simulink model "UART"  (R2020a)
settings: Solver=VariableStepAuto  StartTime=0.0  StopTime=10.0  RelTol=1e-3
libraries: modelsimlib x2, simulink x1
settings Model: Creator=ADMIN  LastModifiedBy=ADMIN

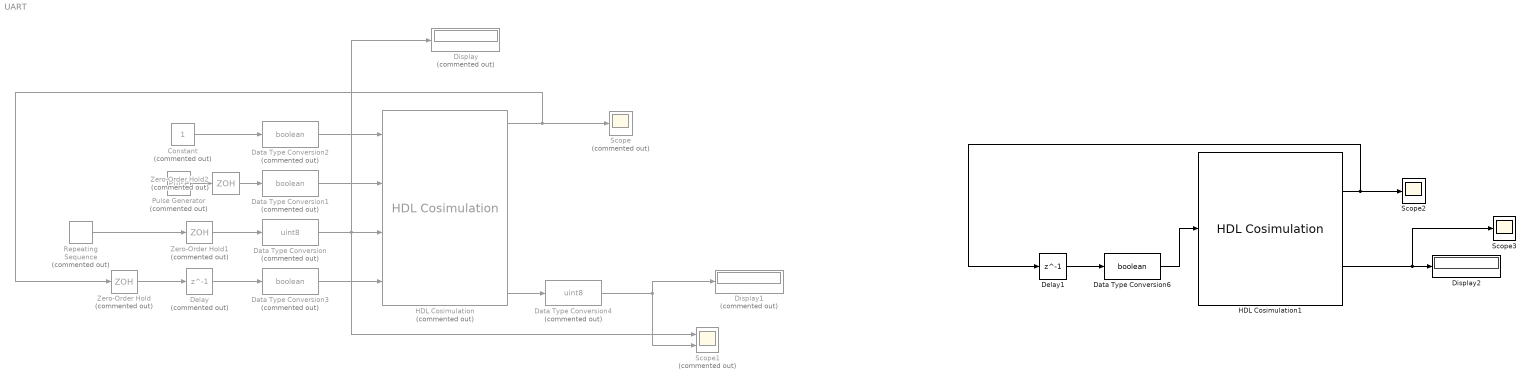
== system UART ==
  Constant : Constant  Commented=on
  Data Type Conversion : DataTypeConversion  Commented=on  OutDataTypeStr=uint8
  Data Type Conversion1 : DataTypeConversion  Commented=on  OutDataTypeStr=boolean
  Data Type Conversion2 : DataTypeConversion  Commented=on  OutDataTypeStr=boolean
  Data Type Conversion3 : DataTypeConversion  Commented=on  OutDataTypeStr=boolean
  Data Type Conversion4 : DataTypeConversion  Commented=on  OutDataTypeStr=uint8
  Data Type Conversion6 : DataTypeConversion  OutDataTypeStr=boolean
  Delay : Delay  Commented=on  DelayLength=1  SampleTime=2e-8
  Delay1 : Delay  DelayLength=1  SampleTime=2e-8
  Display : Display  Commented=on
      settings: Format=binary (Stored Integer)
  Display1 : Display  Commented=on
      settings: Format=binary (Stored Integer)
  Display2 : Display
      settings: Format=binary (Stored Integer)
  HDL Cosimulation : modelsimlib/HDL Cosimulation  Commented=on  PortPaths=/uart/RST_N;/uart/TX_ENA;/uart/TX_DATA;/uart/TX;/uart/TX_BUSY;/uart/TX_DONE;/uart/RX;/uart/RX_BUSY;/uart/RX_ERROR;/uart/RX_DATA  PortModes=[1 1 1 2 2 2 1 2 2 2 ]  PortTimes=[-1,-1,-1,2e-8,2e-8,2e-8,-1,2e-8,2e-8,2e-8]  PortSigns=[-1 -1 -1 -1 -1 -1 -1 -1 -1 -1 ]  PortFracLengths=[0,0,0,0,0,0,0,0,0,0]  CommLocal=on  CommSharedMemory=on  CommPortNumber=4449  CommShowInfo=on  ClockPaths=/uart/CLK  ClockModes=[2 ]  ClockTimes=[2e-8]  TclPreSimCommand="puts \"Running Simulink Cosimulation block.\""  TclPostSimCommand="puts \"done\""  TimingMode=s  TimingScaleFactor=1  idxCellArray={'UNUSED_VAR'}  CosimBypass=Full Simulation  AllowDirectFeedthrough=on  ProductName=EDA Simulator Link MQ  RunAutoTimescale=off  HdlClocks=0  PreRunTime=0  PreRunTimeUnit=ns
      settings: SourceProductBaseCode=ES
  HDL Cosimulation1 : modelsimlib/HDL Cosimulation  PortPaths=/transfer/TX;/transfer/RX;/transfer/RX_DATA  PortModes=[2 1 2 ]  PortTimes=[2e-8,-1,2e-8]  PortSigns=[-1 -1 -1 ]  PortFracLengths=[0,0,0]  CommLocal=on  CommSharedMemory=on  CommPortNumber=4449  CommShowInfo=on  ClockPaths=/transfer/CLK  ClockModes=[2 ]  ClockTimes=[2e-8]  TclPreSimCommand="puts \"Running Simulink Cosimulation block.\""  TclPostSimCommand="puts \"done\""  TimingMode=s  TimingScaleFactor=1  idxCellArray={'UNUSED_VAR'}  CosimBypass=Full Simulation  AllowDirectFeedthrough=on  ProductName=EDA Simulator Link MQ  RunAutoTimescale=off  HdlClocks=0  PreRunTime=0  PreRunTimeUnit=ns
      settings: SourceProductBaseCode=ES
  Pulse Generator : DiscretePulseGenerator  Commented=on  PulseType=Time based  Period=0.001
  Repeating Sequence : simulink/Sources/Repeating Sequence  Commented=on  rep_seq_t=[0 0.2]  rep_seq_y=[0 255]
  Scope : Scope  Commented=on
  Scope1 : Scope  Commented=on  NumInputPorts=2
  Scope2 : Scope
  Scope3 : Scope
  Zero-Order Hold : ZeroOrderHold  Commented=on  SampleTime=2e-8
  Zero-Order Hold1 : ZeroOrderHold  Commented=on  SampleTime=1e-3
  Zero-Order Hold2 : ZeroOrderHold  Commented=on  SampleTime=2e-8
  wires:
  Constant/1 -> Data Type Conversion2/1
  Pulse Generator/1 -> Zero-Order Hold2/1
  Repeating Sequence/1 -> Zero-Order Hold1/1
  HDL Cosimulation/1 -> Zero-Order Hold/1, Scope/1
  Data Type Conversion1/1 -> HDL Cosimulation/2
  Data Type Conversion2/1 -> HDL Cosimulation/1
  Data Type Conversion3/1 -> HDL Cosimulation/4
  Zero-Order Hold/1 -> Delay/1
  Delay/1 -> Data Type Conversion3/1
  HDL Cosimulation/6 -> Data Type Conversion4/1
  Zero-Order Hold1/1 -> Data Type Conversion/1
  Data Type Conversion/1 -> Scope1/1, Display/1, HDL Cosimulation/3
  Data Type Conversion4/1 -> Display1/1, Scope1/2
  Zero-Order Hold2/1 -> Data Type Conversion1/1
  Delay1/1 -> Data Type Conversion6/1
  HDL Cosimulation1/1 -> Delay1/1, Scope2/1
  Data Type Conversion6/1 -> HDL Cosimulation1/1
  HDL Cosimulation1/2 -> Scope3/1, Display2/1
